simulink model "PCV Mode"  (R2025a)
settings: Solver=VariableStepAuto  StartTime=0.0  StopTime=60  RelTol=1e-3
settings Model: Creator=fatihtalay  LastModifiedBy=fatihtalay

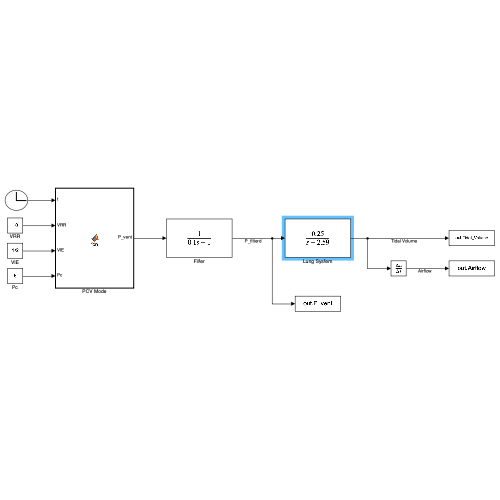
[thumbnail: Simulink's stored preview of the top-level diagram]
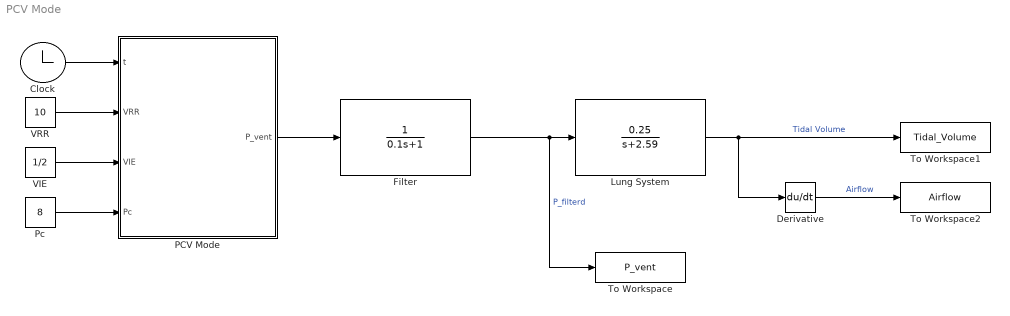
== system PCV Mode ==
  Clock : Clock
  Derivative : Derivative
  Filter : TransferFcn  Denominator=[0.1 1]
  Lung System : TransferFcn  Numerator=[0.25]  Denominator=[1 2.59]
  PCV Mode : MATLAB Function  TreatAsAtomicUnit=on
  Pc : Constant  Value=8
  To Workspace : ToWorkspace  VariableName=P_vent  SaveFormat=Timeseries  SampleTime=-1
  To Workspace1 : ToWorkspace  VariableName=Tidal_Volume  SaveFormat=Timeseries  SampleTime=-1
  To Workspace2 : ToWorkspace  VariableName=Airflow  SaveFormat=Timeseries  SampleTime=-1
  VIE : Constant  Value=1/2
  VRR : Constant  Value=10
  wires:
  Lung System/1 -> To Workspace1/1, Derivative/1  "Tidal Volume"
  Derivative/1 -> To Workspace2/1  "Airflow"
  VRR/1 -> PCV Mode/2(VRR)
  VIE/1 -> PCV Mode/3(VIE)
  Pc/1 -> PCV Mode/4(Pc)
  Clock/1 -> PCV Mode/1(t)
  Filter/1 -> To Workspace/1, Lung System/1  "P_filterd"
  PCV Mode/1(P_vent) -> Filter/1

== matlab function PCV Mode/PCV Mode ==
  data: t input; VRR input; P_vent output; VIE input; Pc input
function P_vent = fcn(t, VRR, VIE, Pc)

T = 60/ VRR ;
TI = T * VIE /(1+ VIE ) ;

P_sq = Pc * (mod(t, T) <= TI);

P_vent = P_sq;
